simulink model "vicon_hexatilted_read"  (R2023a)
settings: Solver=ode4  StartTime=0.0  StopTime=tf  FixedStep=0.01  RelTol=1e-3
values from neighbouring files (symbols this model uses):
  s = saveObjectImpl@matlab.System(obj)    [movingAverageFilter.m]
  sigmanoise = 0.0000001    (= 1e-07)    [vicon_hexatilted.m]
undefined symbols (not defined in the file or in its folder): X, Y, Z
libraries: sm_lib x15, nesl_utility x11, commchan3 x4, aerolibutil x4, sharedtransform x3, robotlib x3, dspstat3 x1
settings Model: Creator=main  LastModifiedBy=Dell

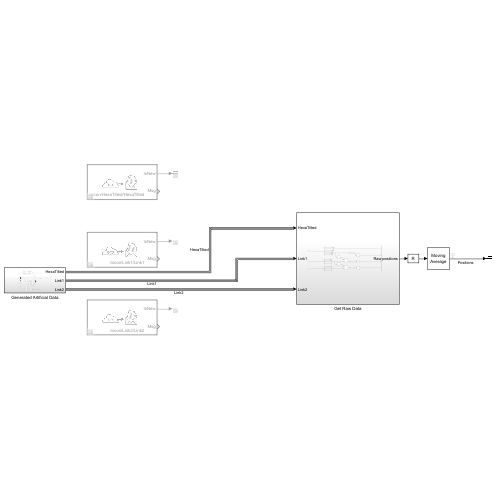
[thumbnail: Simulink's stored preview of the top-level diagram]
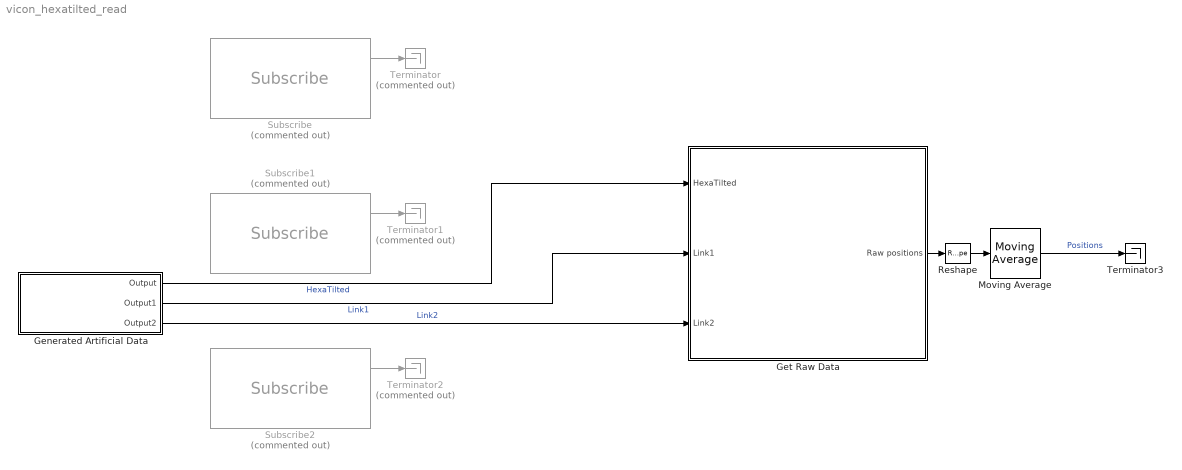
== system vicon_hexatilted_read ==
  Generated Artificial Data : Subsystem
  Get Raw Data : Subsystem
  Moving Average : dspstat3/Moving Average  Method=Sliding window  ForgettingFactorPort=off  SpecifyWindowLength=on  WindowLength=4  OverlapLength=3  AllowArbitraryInputLength=off  ForgettingFactor=0.9  SimulateUsing=Code generation
  Reshape : Reshape  OutputDimensionality=Customize  OutputDimensions=[1,8]
  Subscribe : robotlib/Subscribe  Commented=on  topicSource=Specify your own  topic=/vicon/HexaTilted/HexaTilted  messageType=geometry_msgs/TransformStamped  SampleTime=-1  legacyBusStruct=off  messageQueueLength=1
  Subscribe1 : robotlib/Subscribe  Commented=on  topicSource=Specify your own  topic=/vicon/Link1/Link1  messageType=geometry_msgs/TransformStamped  SampleTime=-1  legacyBusStruct=off  messageQueueLength=1
  Subscribe2 : robotlib/Subscribe  Commented=on  topicSource=Specify your own  topic=/vicon/Link2/Link2  messageType=geometry_msgs/TransformStamped  SampleTime=-1  legacyBusStruct=off  messageQueueLength=1
  Terminator : Terminator  Commented=on
  Terminator1 : Terminator  Commented=on
  Terminator2 : Terminator  Commented=on
  Terminator3 : Terminator
  wires:
  Subscribe/1 -> Terminator/1
  Subscribe1/1 -> Terminator1/1
  Subscribe2/1 -> Terminator2/1
  Generated Artificial Data/1(Output) -> Get Raw Data/1(HexaTilted)  "HexaTilted"
  Generated Artificial Data/2(Output1) -> Get Raw Data/2(Link1)  "Link1"
  Generated Artificial Data/3(Output2) -> Get Raw Data/3(Link2)  "Link2"
  Get Raw Data/1(Raw positions) -> Reshape/1
  Reshape/1 -> Moving Average/1
  Moving Average/1 -> Terminator3/1  "Positions"

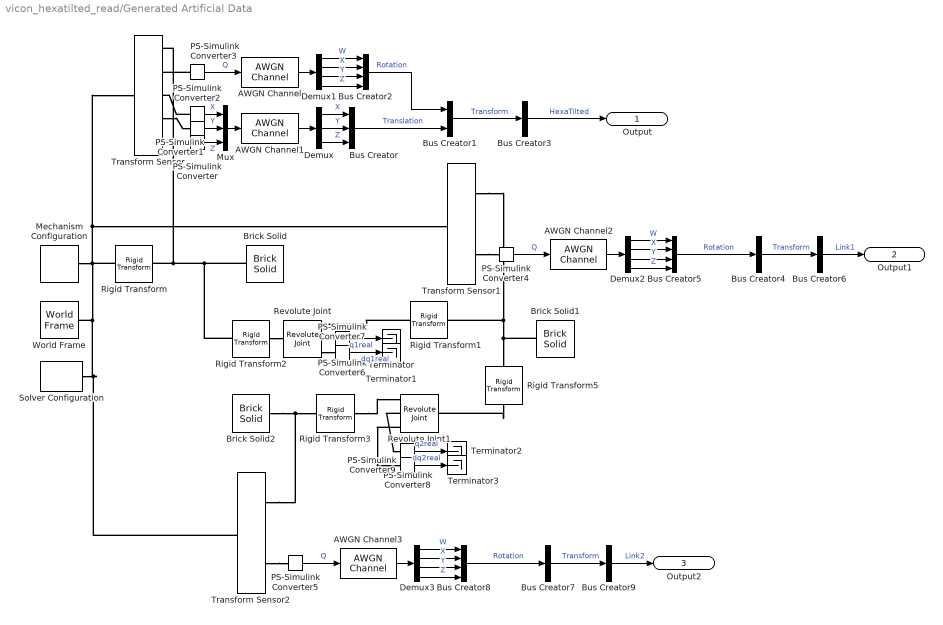
== system vicon_hexatilted_read/Generated Artificial Data ==
  AWGN Channel{,1..3} (4 alike) : commchan3/AWGN Channel  LegacyMode=off  NoiseMethod=Variance  noiseMode="Signal to noise ratio  (SNR)"  EbNo=10  EsNo=10  SNR=10  BitsPerSymbol=1  SignalPower=1  SamplesPerSymbol=1  SymbolPeriod=1  VarianceSource=Parameter  Variance=sigmanoise  RandomStream=Global stream  Seed=67  SimulateUsing=Code generation
  Brick Solid : sm_lib/Body Elements/Brick Solid  GraphicAmbientColor=[0.15 0.15 0.15 1.0]  BasedOnType=Density  BrickDimensions=[0.25 0.25 0.01]  BrickDimensionsUnits=m  CenterOfMass=[0 0 0]  CenterOfMassUnits=m  GraphicDiffuseColor=[0.5 0.5 0.5]  Density=1000  DensityUnits=kg/m^3  DoExposeReferenceFrame=on  GraphicEmissiveColor=[0.0 0.0 0.0 1.0]  ExportEntireGeometry=off  SerializedFrames=<Frames/>  MarkerShape=Sphere  MarkerSize=10  GraphicType=FromGeometry  InertiaType=CalculateFromGeometry  Mass=1  MassUnits=kg  MomentsOfInertia=[1 1 1]  MomentsOfInertiaUnits=kg*m^2  GraphicOpacity=1.0  ProductsOfInertia=[0 0 0]  ProductsOfInertiaUnits=kg*m^2  GraphicShininess=75  GraphicSpecularColor=[0.5 0.5 0.5 1.0]  GraphicVisPropType=SimpleVisualProperties
  Brick Solid1 : sm_lib/Body Elements/Brick Solid  GraphicAmbientColor=[0.15 0.15 0.15 1.0]  BasedOnType=Density  BrickDimensions=[0.01 0.01 0.15]  BrickDimensionsUnits=m  CenterOfMass=[0 0 0]  CenterOfMassUnits=m  GraphicDiffuseColor=[0.5 0.5 0.5]  Density=1000  DensityUnits=kg/m^3  DoExposeReferenceFrame=on  GraphicEmissiveColor=[0.0 0.0 0.0 1.0]  ExportEntireGeometry=off  SerializedFrames=<Frames/>  MarkerShape=Sphere  MarkerSize=10  GraphicType=FromGeometry  InertiaType=CalculateFromGeometry  Mass=1  MassUnits=kg  MomentsOfInertia=[1 1 1]  MomentsOfInertiaUnits=kg*m^2  GraphicOpacity=1.0  ProductsOfInertia=[0 0 0]  ProductsOfInertiaUnits=kg*m^2  GraphicShininess=75  GraphicSpecularColor=[0.5 0.5 0.5 1.0]  GraphicVisPropType=SimpleVisualProperties
  Brick Solid2 : sm_lib/Body Elements/Brick Solid  GraphicAmbientColor=[0.15 0.15 0.15 1.0]  BasedOnType=Density  BrickDimensions=[0.01 0.01 0.15]  BrickDimensionsUnits=m  CenterOfMass=[0 0 0]  CenterOfMassUnits=m  GraphicDiffuseColor=[0.5 0.5 0.5]  Density=1000  DensityUnits=kg/m^3  DoExposeReferenceFrame=on  GraphicEmissiveColor=[0.0 0.0 0.0 1.0]  ExportEntireGeometry=off  SerializedFrames=<Frames/>  MarkerShape=Sphere  MarkerSize=10  GraphicType=FromGeometry  InertiaType=CalculateFromGeometry  Mass=1  MassUnits=kg  MomentsOfInertia=[1 1 1]  MomentsOfInertiaUnits=kg*m^2  GraphicOpacity=1.0  ProductsOfInertia=[0 0 0]  ProductsOfInertiaUnits=kg*m^2  GraphicShininess=75  GraphicSpecularColor=[0.5 0.5 0.5 1.0]  GraphicVisPropType=SimpleVisualProperties
  Bus Creator : BusCreator  Inputs=3
  Bus Creator1 : BusCreator  Inputs=2
  Bus Creator2 : BusCreator  Inputs=4
  Bus Creator{3..4,6..7,9} (5 alike) : BusCreator  Inputs=1
  Bus Creator5 : BusCreator  Inputs=4
  Bus Creator8 : BusCreator  Inputs=4
  Demux : Demux  Outputs=3
  Demux1 : Demux
  Demux2 : Demux
  Demux3 : Demux
  Mechanism Configuration : sm_lib/Utilities/Mechanism Configuration  UniformGravity=Constant  GravityVector=[0 0 -9.80665]  GravityVectorUnits=m/s^2  LinearizationDelta=0.001  JointModeTransitionNonlinearIterations=2
  Mux : Mux  Inputs=3
  PS-Simulink Converter{,1..9} (10 alike) : nesl_utility/PS-Simulink Converter  PhysicalDomain=network_engine_domain  SubClassName=ps_output  LeftPortType=input  RightPortType=output  PseudoPeriodic=off  Frequencies=[]  VectorFormat=inherit  Unit=inherit  AffineConversion=off
  Revolute Joint : sm_lib/Joints/Revolute Joint  JointMode=Normal  SenseConstraintForce=off  SenseConstraintForceX=off  SenseConstraintForceY=off  SenseConstraintForceZ=off  SenseConstraintTorque=off  SenseConstraintTorqueX=off  SenseConstraintTorqueY=off  SenseConstraintTorqueZ=off  SenseTotalForce=off  SenseTotalForceX=off  SenseTotalForceY=off  SenseTotalForceZ=off  SenseTotalTorque=off  SenseTotalTorqueX=off  SenseTotalTorqueY=off  SenseTotalTorqueZ=off  CompositeWrenchDir=FollowerOnBase  CompositeWrenchFrame=BaseFrame  EquilibriumPosition=0  EquilibriumPositionUnits=deg  SpringStiffness=0  SpringStiffnessUnits=N*m/deg  DampingCoefficient=0  DampingCoefficientUnits=N*m/(deg/s)  TorqueActuationMode=NoTorque  MotionActuationMode=ComputedMotion  SensePosition=on  SenseVelocity=on  SenseAcceleration=off  SenseTorqueForce=off  SenseLowerLimitTorqueForce=off  SenseUpperLimitTorqueForce=off  LowerLimitSpecify=off  LowerLimitBound=-90  LowerLimitBoundUnits=deg  LowerLimitStiffness=1e4  LowerLimitStiffnessUnits=N*m/deg  LowerLimitDamping=10  LowerLimitDampingUnits=N*m/(deg/s)  LowerLimitTransitionRegionWidth=0.1  LowerLimitTransitionRegionWidthUnits=deg  UpperLimitSpecify=off  UpperLimitBound=90  UpperLimitBoundUnits=deg  UpperLimitStiffness=1e4  UpperLimitStiffnessUnits=N*m/deg  UpperLimitDamping=10  UpperLimitDampingUnits=N*m/(deg/s)  UpperLimitTransitionRegionWidth=0.1  UpperLimitTransitionRegionWidthUnits=deg  PositionTargetSpecify=on  PositionTargetPriority=High  PositionTargetValue=0.5  PositionTargetValueUnits=deg  VelocityTargetSpecify=off  VelocityTargetPriority=High  VelocityTargetValue=0  VelocityTargetValueUnits=deg/s
  Revolute Joint1 : sm_lib/Joints/Revolute Joint  JointMode=Normal  SenseConstraintForce=off  SenseConstraintForceX=off  SenseConstraintForceY=off  SenseConstraintForceZ=off  SenseConstraintTorque=off  SenseConstraintTorqueX=off  SenseConstraintTorqueY=off  SenseConstraintTorqueZ=off  SenseTotalForce=off  SenseTotalForceX=off  SenseTotalForceY=off  SenseTotalForceZ=off  SenseTotalTorque=off  SenseTotalTorqueX=off  SenseTotalTorqueY=off  SenseTotalTorqueZ=off  CompositeWrenchDir=FollowerOnBase  CompositeWrenchFrame=BaseFrame  EquilibriumPosition=0  EquilibriumPositionUnits=deg  SpringStiffness=0  SpringStiffnessUnits=N*m/deg  DampingCoefficient=0  DampingCoefficientUnits=N*m/(deg/s)  TorqueActuationMode=NoTorque  MotionActuationMode=ComputedMotion  SensePosition=on  SenseVelocity=on  SenseAcceleration=off  SenseTorqueForce=off  SenseLowerLimitTorqueForce=off  SenseUpperLimitTorqueForce=off  LowerLimitSpecify=off  LowerLimitBound=-90  LowerLimitBoundUnits=deg  LowerLimitStiffness=1e4  LowerLimitStiffnessUnits=N*m/deg  LowerLimitDamping=10  LowerLimitDampingUnits=N*m/(deg/s)  LowerLimitTransitionRegionWidth=0.1  LowerLimitTransitionRegionWidthUnits=deg  UpperLimitSpecify=off  UpperLimitBound=90  UpperLimitBoundUnits=deg  UpperLimitStiffness=1e4  UpperLimitStiffnessUnits=N*m/deg  UpperLimitDamping=10  UpperLimitDampingUnits=N*m/(deg/s)  UpperLimitTransitionRegionWidth=0.1  UpperLimitTransitionRegionWidthUnits=deg  PositionTargetSpecify=on  PositionTargetPriority=High  PositionTargetValue=1  PositionTargetValueUnits=deg  VelocityTargetSpecify=off  VelocityTargetPriority=High  VelocityTargetValue=0  VelocityTargetValueUnits=deg/s
  Rigid Transform : sm_lib/Frames and Transforms/Rigid Transform  TranslationMethod=Cartesian  TranslationStandardOffset=0  TranslationStandardOffsetUnits=m  TranslationStandardAxis=+Z  TranslationCartesianOffset=[0 0 1]  TranslationCartesianOffsetUnits=m  TranslationROffset=0  TranslationROffsetUnits=m  TranslationZOffset=0  TranslationZOffsetUnits=m  TranslationThetaOffset=0  TranslationThetaOffsetUnits=deg  RotationMethod=None  RotationAngleUnits=deg  RotationStandardAxis=+Z  RotationAngle=0.0  RotationArbitraryAxis=[0 0 1]  FollAlignAxisA=+X  BaseAlignAxisA=+Y  FollAlignAxisB=+Y  BaseAlignAxisB=+Z  RotationSequenceAxes=FollowerAxes  RotationSequence=XYX  RotationSequenceAngles=[0 0 0]  RotationSequenceAnglesUnits=deg  RotationMatrix=[1 0 0; 0 1 0; 0 0 1]  Quaternion=[1 0 0 0]
  Rigid Transform1 : sm_lib/Frames and Transforms/Rigid Transform  TranslationMethod=Cartesian  TranslationStandardOffset=0  TranslationStandardOffsetUnits=m  TranslationStandardAxis=+Z  TranslationCartesianOffset=[0 0 0.075]  TranslationCartesianOffsetUnits=m  TranslationROffset=0  TranslationROffsetUnits=m  TranslationZOffset=0  TranslationZOffsetUnits=m  TranslationThetaOffset=0  TranslationThetaOffsetUnits=deg  RotationMethod=StandardAxis  RotationAngleUnits=deg  RotationStandardAxis=+Y  RotationAngle=90  RotationArbitraryAxis=[0 0 1]  FollAlignAxisA=+X  BaseAlignAxisA=+Y  FollAlignAxisB=+Y  BaseAlignAxisB=+Z  RotationSequenceAxes=FollowerAxes  RotationSequence=XYX  RotationSequenceAngles=[0 0 0]  RotationSequenceAnglesUnits=deg  RotationMatrix=[1 0 0; 0 1 0; 0 0 1]  Quaternion=[1 0 0 0]
  Rigid Transform2 : sm_lib/Frames and Transforms/Rigid Transform  TranslationMethod=None  TranslationStandardOffset=0  TranslationStandardOffsetUnits=m  TranslationStandardAxis=+Z  TranslationCartesianOffset=[0 0 0]  TranslationCartesianOffsetUnits=m  TranslationROffset=0  TranslationROffsetUnits=m  TranslationZOffset=0  TranslationZOffsetUnits=m  TranslationThetaOffset=0  TranslationThetaOffsetUnits=deg  RotationMethod=StandardAxis  RotationAngleUnits=deg  RotationStandardAxis=+Y  RotationAngle=90  RotationArbitraryAxis=[0 0 1]  FollAlignAxisA=+X  BaseAlignAxisA=+Y  FollAlignAxisB=+Y  BaseAlignAxisB=+Z  RotationSequenceAxes=FollowerAxes  RotationSequence=XYX  RotationSequenceAngles=[0 0 0]  RotationSequenceAnglesUnits=deg  RotationMatrix=[1 0 0; 0 1 0; 0 0 1]  Quaternion=[1 0 0 0]
  Rigid Transform3 : sm_lib/Frames and Transforms/Rigid Transform  TranslationMethod=Cartesian  TranslationStandardOffset=0  TranslationStandardOffsetUnits=m  TranslationStandardAxis=+Z  TranslationCartesianOffset=[0 0 0.075]  TranslationCartesianOffsetUnits=m  TranslationROffset=0  TranslationROffsetUnits=m  TranslationZOffset=0  TranslationZOffsetUnits=m  TranslationThetaOffset=0  TranslationThetaOffsetUnits=deg  RotationMethod=StandardAxis  RotationAngleUnits=deg  RotationStandardAxis=+Y  RotationAngle=90  RotationArbitraryAxis=[0 0 1]  FollAlignAxisA=+X  BaseAlignAxisA=+Y  FollAlignAxisB=+Y  BaseAlignAxisB=+Z  RotationSequenceAxes=FollowerAxes  RotationSequence=XYX  RotationSequenceAngles=[0 0 0]  RotationSequenceAnglesUnits=deg  RotationMatrix=[1 0 0; 0 1 0; 0 0 1]  Quaternion=[1 0 0 0]
  Rigid Transform5 : sm_lib/Frames and Transforms/Rigid Transform  TranslationMethod=Cartesian  TranslationStandardOffset=0  TranslationStandardOffsetUnits=m  TranslationStandardAxis=+Z  TranslationCartesianOffset=[0 0 -0.075]  TranslationCartesianOffsetUnits=m  TranslationROffset=0  TranslationROffsetUnits=m  TranslationZOffset=0  TranslationZOffsetUnits=m  TranslationThetaOffset=0  TranslationThetaOffsetUnits=deg  RotationMethod=StandardAxis  RotationAngleUnits=deg  RotationStandardAxis=+Y  RotationAngle=90  RotationArbitraryAxis=[0 0 1]  FollAlignAxisA=+X  BaseAlignAxisA=+Y  FollAlignAxisB=+Y  BaseAlignAxisB=+Z  RotationSequenceAxes=FollowerAxes  RotationSequence=XYX  RotationSequenceAngles=[0 0 0]  RotationSequenceAnglesUnits=deg  RotationMatrix=[1 0 0; 0 1 0; 0 0 1]  Quaternion=[1 0 0 0]
  Solver Configuration : nesl_utility/Solver Configuration  PhysicalDomain=network_engine_domain  SubClassName=solver  LeftPortType=input  RightPortType=generic  Tones=[]  Harmonics=[]  SimulateNoise=off  Profile=off  UseLocalSampling=off  EnableSwitchedLinearOptims=on  FrequencyDomain=off  UseCCode=off  RelTol=0.001  AbsTol=0.001  MinStep=1e-09  ToWorkspace=off  RevertToSquareIcSolve=off  NumHomotopyIterations=100  PhasorMode=off  PhasorModeNumHarmonics=1  ConsistencySolver=NEWTON_XTOL_AFTER_FTOL  IndexReductionMethod=DerivativeReplacement  DoDC=off  ResidualTolerance=1e-09  ConsistencyTolSource=GLOBAL  ConsistencyAbsTol=0.001  ConsistencyRelTol=0.001  ConsistencyTolFactor=0.001  UseLocalSolver=off  LocalSolverChoice=NE_BACKWARD_EULER_ADVANCER  ResolveIndetEquations=on  FunctionEvalNumThread=1  LocalSolverSampleTime=0.001  DoFixedCost=off  MaxNonlinIter=3  MaxModeIter=2  ComputeImpulses=off  ImpulseIterations=2  LinearAlgebra=auto  LinearAlgebraNumThread=0  EquationFormulation=NE_TIME_EF  DelaysMemoryBudget=1024  AutomaticFiltering=on  FilteringTimeConstant=0.001  PartitionStorageMethod=AS_NEEDED  PartitionMemoryBudget=1024  PartitionMethod=ROBUST
  Terminator{,1..3} (4 alike) : Terminator
  Transform Sensor : sm_lib/Frames and Transforms/Transform Sensor  MeasurementFrame=World  RotationSequence=XYX  SenseAngle=off  SenseAxis=off  SenseQ=on  SenseR=off  SenseRotationSequence=off  SenseOmegaX=off  SenseOmegaY=off  SenseOmegaZ=off  SenseQDot=off  SenseRDot=off  SenseRotationSequenceDot=off  SenseAlphaX=off  SenseAlphaY=off  SenseAlphaZ=off  SenseQDDot=off  SenseRDDot=off  SenseX=on  SenseY=on  SenseZ=on  SenseRad=off  SenseAzim=off  SenseDist=off  SenseInc=off  SenseXDot=off  SenseYDot=off  SenseZDot=off  SenseRadDot=off  SenseAzimDot=off  SenseDistDot=off  SenseIncDot=off  SenseXDDot=off  SenseYDDot=off  SenseZDDot=off  SenseRadDDot=off  SenseAzimDDot=off  SenseDistDDot=off  SenseIncDDot=off
  Transform Sensor1 : sm_lib/Frames and Transforms/Transform Sensor  MeasurementFrame=World  RotationSequence=XYX  SenseAngle=off  SenseAxis=off  SenseQ=on  SenseR=off  SenseRotationSequence=off  SenseOmegaX=off  SenseOmegaY=off  SenseOmegaZ=off  SenseQDot=off  SenseRDot=off  SenseRotationSequenceDot=off  SenseAlphaX=off  SenseAlphaY=off  SenseAlphaZ=off  SenseQDDot=off  SenseRDDot=off  SenseX=off  SenseY=off  SenseZ=off  SenseRad=off  SenseAzim=off  SenseDist=off  SenseInc=off  SenseXDot=off  SenseYDot=off  SenseZDot=off  SenseRadDot=off  SenseAzimDot=off  SenseDistDot=off  SenseIncDot=off  SenseXDDot=off  SenseYDDot=off  SenseZDDot=off  SenseRadDDot=off  SenseAzimDDot=off  SenseDistDDot=off  SenseIncDDot=off
  Transform Sensor2 : sm_lib/Frames and Transforms/Transform Sensor  MeasurementFrame=World  RotationSequence=XYX  SenseAngle=off  SenseAxis=off  SenseQ=on  SenseR=off  SenseRotationSequence=off  SenseOmegaX=off  SenseOmegaY=off  SenseOmegaZ=off  SenseQDot=off  SenseRDot=off  SenseRotationSequenceDot=off  SenseAlphaX=off  SenseAlphaY=off  SenseAlphaZ=off  SenseQDDot=off  SenseRDDot=off  SenseX=off  SenseY=off  SenseZ=off  SenseRad=off  SenseAzim=off  SenseDist=off  SenseInc=off  SenseXDot=off  SenseYDot=off  SenseZDot=off  SenseRadDot=off  SenseAzimDot=off  SenseDistDot=off  SenseIncDot=off  SenseXDDot=off  SenseYDDot=off  SenseZDDot=off  SenseRadDDot=off  SenseAzimDDot=off  SenseDistDDot=off  SenseIncDDot=off
  World Frame : sm_lib/Frames and Transforms/World Frame
  Output : Outport
  Output1 : Outport  Port=2
  Output2 : Outport  Port=3
  wires:
  Demux1/3 -> Bus Creator2/3  "Y"
  Bus Creator1/1 -> Bus Creator3/1  "Transform"
  Bus Creator3/1 -> Output/1  "HexaTilted"
  Bus Creator/1 -> Bus Creator1/2  "Translation"
  Demux1/4 -> Bus Creator2/4  "Z"
  Demux1/1 -> Bus Creator2/1  "W"
  Bus Creator2/1 -> Bus Creator1/1  "Rotation"
  Demux1/2 -> Bus Creator2/2  "X"
  PS-Simulink Converter3/1 -> AWGN Channel/1  "Q"
  AWGN Channel/1 -> Demux1/1
  PS-Simulink Converter2/1 -> Mux/1  "X"
  PS-Simulink Converter1/1 -> Mux/2  "Y"
  PS-Simulink Converter/1 -> Mux/3  "Z"
  Mux/1 -> AWGN Channel1/1
  AWGN Channel1/1 -> Demux/1
  Demux/1 -> Bus Creator/1  "X"
  Demux/2 -> Bus Creator/2  "Y"
  Demux/3 -> Bus Creator/3  "Z"
  PS-Simulink Converter4/1 -> AWGN Channel2/1  "Q"
  Bus Creator5/1 -> Bus Creator4/1  "Rotation"
  AWGN Channel2/1 -> Demux2/1
  Demux2/4 -> Bus Creator5/4  "Z"
  Demux2/1 -> Bus Creator5/1  "W"
  Demux2/3 -> Bus Creator5/3  "Y"
  Demux2/2 -> Bus Creator5/2  "X"
  Bus Creator4/1 -> Bus Creator6/1  "Transform"
  Bus Creator6/1 -> Output1/1  "Link1"
  Demux3/2 -> Bus Creator8/2  "X"
  Demux3/1 -> Bus Creator8/1  "W"
  Demux3/3 -> Bus Creator8/3  "Y"
  PS-Simulink Converter5/1 -> AWGN Channel3/1  "Q"
  Bus Creator8/1 -> Bus Creator7/1  "Rotation"
  Bus Creator9/1 -> Output2/1  "Link2"
  AWGN Channel3/1 -> Demux3/1
  Bus Creator7/1 -> Bus Creator9/1  "Transform"
  Demux3/4 -> Bus Creator8/4  "Z"
  PS-Simulink Converter6/1 -> Terminator/1  "q1real"
  PS-Simulink Converter7/1 -> Terminator1/1  "dq1real"
  PS-Simulink Converter9/1 -> Terminator3/1  "dq2real"
  PS-Simulink Converter8/1 -> Terminator2/1  "q2real"
  connections:
  Brick Solid/RConn1 -- Transform Sensor/RConn1 -- Rigid Transform/RConn1 -- Rigid Transform2/LConn1
  Rigid Transform5/RConn1 -- Revolute Joint1/LConn1
  Rigid Transform3/RConn1 -- Revolute Joint1/RConn1
  Solver Configuration/RConn1 -- Transform Sensor2/LConn1 -- Rigid Transform/LConn1 -- Mechanism Configuration/RConn1 -- Transform Sensor/LConn1 -- Transform Sensor1/LConn1 -- World Frame/RConn1
  Brick Solid1/RConn1 -- Transform Sensor1/RConn1 -- Rigid Transform1/LConn1 -- Rigid Transform5/LConn1
  PS-Simulink Converter3/LConn1 -- Transform Sensor/RConn2
  PS-Simulink Converter2/LConn1 -- Transform Sensor/RConn3
  Rigid Transform1/RConn1 -- Revolute Joint/RConn1
  Transform Sensor/RConn4 -- PS-Simulink Converter1/LConn1
  Brick Solid2/RConn1 -- Transform Sensor2/RConn1 -- Rigid Transform3/LConn1
  Rigid Transform2/RConn1 -- Revolute Joint/LConn1
  PS-Simulink Converter/LConn1 -- Transform Sensor/RConn5
  Transform Sensor1/RConn2 -- PS-Simulink Converter4/LConn1
  Transform Sensor2/RConn2 -- PS-Simulink Converter5/LConn1
  Revolute Joint/RConn2 -- PS-Simulink Converter6/LConn1
  Revolute Joint/RConn3 -- PS-Simulink Converter7/LConn1
  Revolute Joint1/RConn2 -- PS-Simulink Converter8/LConn1
  Revolute Joint1/RConn3 -- PS-Simulink Converter9/LConn1

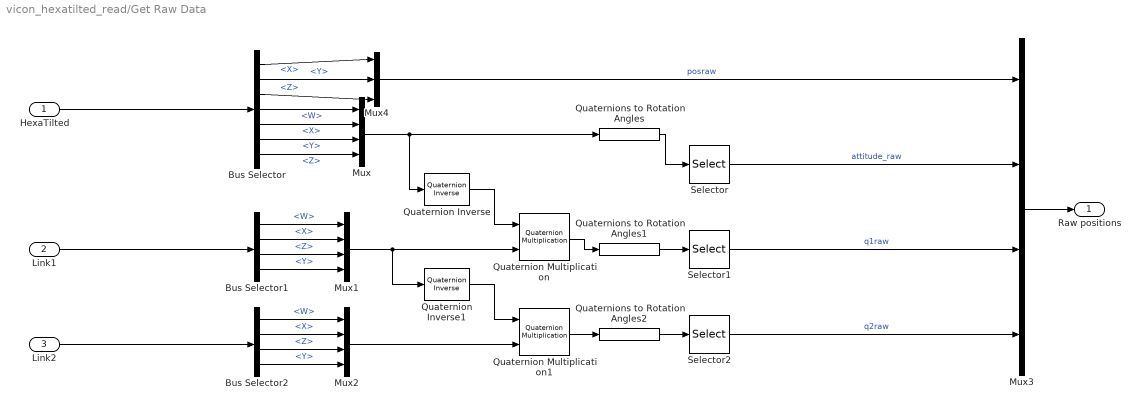
== system vicon_hexatilted_read/Get Raw Data ==
  HexaTilted : Inport
  Link1 : Inport  Port=2
  Link2 : Inport  Port=3
  Bus Selector : BusSelector  OutputSignals=Transform.Translation.X,Transform.Translation.Y,Transform.Translation.Z,Transform.Rotation.W,Transform.Rotation.X,Transform.Rotation.Y,Transform.Rotation.Z
  Bus Selector1 : BusSelector  OutputSignals=Transform.Rotation.W,Transform.Rotation.X,Transform.Rotation.Z,Transform.Rotation.Y
  Bus Selector2 : BusSelector  OutputSignals=Transform.Rotation.W,Transform.Rotation.X,Transform.Rotation.Z,Transform.Rotation.Y
  Mux{,1..3} (4 alike) : Mux
  Mux4 : Mux  Inputs=3
  Quaternion Inverse : aerolibutil/Quaternion Inverse
  Quaternion Inverse1 : aerolibutil/Quaternion Inverse
  Quaternion Multiplication : aerolibutil/Quaternion Multiplication
  Quaternion Multiplication1 : aerolibutil/Quaternion Multiplication
  Quaternions to Rotation Angles : sharedtransform/Quaternions to Rotation Angles  rotationOrder=ZYX  aMode=aMode
  Quaternions to Rotation Angles1 : sharedtransform/Quaternions to Rotation Angles  rotationOrder=ZYX  aMode=aMode
  Quaternions to Rotation Angles2 : sharedtransform/Quaternions to Rotation Angles  rotationOrder=ZYX  aMode=aMode
  Selector : Selector  InputPortWidth=3  IndexOptions=Index vector (dialog)  Indices=3:-1:1  OutputSizes=1
  Selector1 : Selector  InputPortWidth=3  IndexOptions=Index vector (dialog)  Indices=3  OutputSizes=1
  Selector2 : Selector  InputPortWidth=3  IndexOptions=Index vector (dialog)  Indices=3  OutputSizes=1
  Raw positions : Outport
  wires:
  Selector2/1 -> Mux3/4  "q2raw"
  Bus Selector/4 -> Mux/1  "<W>"
  Bus Selector2/2 -> Mux2/2  "<X>"
  Quaternions to Rotation Angles1/1 -> Selector1/1
  Mux1/1 -> Quaternion Inverse1/1, Quaternion Multiplication/2
  Bus Selector1/4 -> Mux1/4  "<Y>"
  Bus Selector2/3 -> Mux2/3  "<Z>"
  Bus Selector/5 -> Mux/2  "<X>"
  Quaternions to Rotation Angles/1 -> Selector/1
  Bus Selector/6 -> Mux/3  "<Y>"
  Mux/1 -> Quaternion Inverse/1, Quaternions to Rotation Angles/1
  Bus Selector1/3 -> Mux1/3  "<Z>"
  Quaternions to Rotation Angles2/1 -> Selector2/1
  Quaternion Multiplication/1 -> Quaternions to Rotation Angles1/1
  Quaternion Multiplication1/1 -> Quaternions to Rotation Angles2/1
  Selector1/1 -> Mux3/3  "q1raw"
  Mux2/1 -> Quaternion Multiplication1/2
  Bus Selector2/1 -> Mux2/1  "<W>"
  Quaternion Inverse/1 -> Quaternion Multiplication/1
  Bus Selector2/4 -> Mux2/4  "<Y>"
  Quaternion Inverse1/1 -> Quaternion Multiplication1/1
  Link2/1 -> Bus Selector2/1
  HexaTilted/1 -> Bus Selector/1
  Bus Selector/7 -> Mux/4  "<Z>"
  Bus Selector1/2 -> Mux1/2  "<X>"
  Bus Selector1/1 -> Mux1/1  "<W>"
  Selector/1 -> Mux3/2  "attitude_raw"
  Link1/1 -> Bus Selector1/1
  Mux4/1 -> Mux3/1  "posraw"
  Bus Selector/1 -> Mux4/1  "<X>"
  Bus Selector/2 -> Mux4/2  "<Y>"
  Bus Selector/3 -> Mux4/3  "<Z>"
  Mux3/1 -> Raw positions/1
